simulink model "kalman_filter"  (Simulink 8.7)
settings: Solver=FixedStepAuto  StartTime=0.0  StopTime=10.0  FixedStep=dt  RelTol=1e-3
values from neighbouring files (symbols this model uses):
  A = [1 dt; 0 1]    [kalman_filter_init.m]
  B = zeros(2, 1)    [kalman_filter_init.m]
  dt = 1/50    (= 0.02)    [kalman_filter_init.m]
  H = eye(2, 2)    [kalman_filter_init.m]
  P0 = Q    [kalman_filter_init.m]
  Q = 0.01*eye(2,2)    [kalman_filter_init.m]
  R = 0.95*eye(2,2)    [kalman_filter_init.m]
  x0 = [0 0]'    [kalman_filter_init.m]
  x_seed = round(abs(rand()*1000))    [kalman_filter_init.m]
  xdot_seed = round(abs(rand()*1000))    [kalman_filter_init.m]
libraries: aerolibnav x2
settings Model: Creator=jason  LastModifiedBy=jason
settings DataIOCC: LimitDataPoints=off  SaveFormat=Dataset
settings DebuggingCC: UnderspecifiedInitializationDetection=Simplified  MergeDetectMultiDrivingBlocksExec=error
settings HardwareCC: ProdBitPerPointer=64  ProdLargestAtomicFloat=Float  ProdIntDivRoundTo=Zero  ProdEndianess=LittleEndian  ProdWordSize=64  ProdHWDeviceType=Intel->x86-64 (Windows64)
settings ModelReferenceCC: PropagateSignalLabelsOutOfModel=on
settings ConfigComp: CovModelRefEnable=off

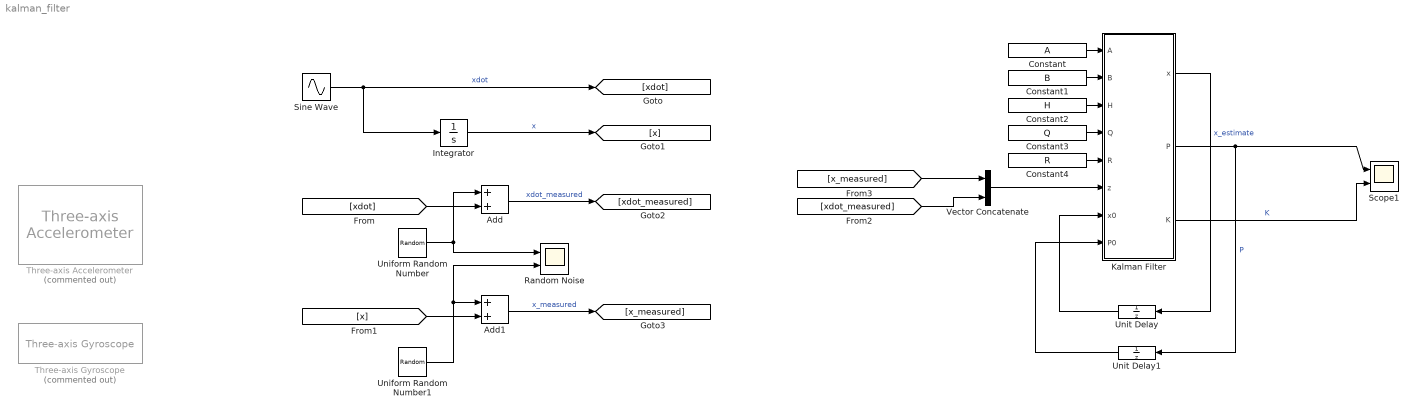
== system kalman_filter ==
  Add : Sum
  Add1 : Sum
  Constant : Constant  Value=A
  Constant1 : Constant  Value=B
  Constant2 : Constant  Value=H
  Constant3 : Constant  Value=Q
  Constant4 : Constant  Value=R
  Integrator : Integrator
  Kalman Filter : MATLAB Function  TreatAsAtomicUnit=on
  Random Noise : Scope  NumInputPorts=2
  Scope1 : Scope  NumInputPorts=2
  Sine Wave : Sin  SampleTime=0
  Three-axis Accelerometer : aerolibnav/Three-axis Accelerometer  Commented=on  units=Metric (MKS)  acc=[0 0 0]  gtype=on  dtype_a=on  w_a=190  z_a=0.707  a_sf_cc=[1 0 0; 0 1 0; 0 0 1]  a_bias=[0 0 0]  a_Ts=0  a_rand=on  a_seeds=[23093 23094 23095]  a_pow=[0.001 0.001 0.001]  a_sat="[-inf  -inf  -inf  inf inf inf]"
  Three-axis Gyroscope : aerolibnav/Three-axis Gyroscope  Commented=on  dtype_g=on  w_g=190  z_g=0.707  g_sf_cc=[1 0 0; 0 1 0; 0 0 1]  g_bias=[0 0 0]  g_sen=[0 0 0]  g_Ts=0  g_rand=on  g_seeds=[23093 23094 23095]  g_pow=[0.0001 0.0001 0.0001]  g_sat="[-inf  -inf  -inf  inf inf inf]"
  Uniform Random Number : UniformRandomNumber  Seed=xdot_seed  SampleTime=dt
  Uniform Random Number1 : UniformRandomNumber  Seed=x_seed  SampleTime=dt
  Unit Delay : UnitDelay  InitialCondition=x0  SampleTime=-1
  Unit Delay1 : UnitDelay  InitialCondition=P0  SampleTime=-1
  Vector Concatenate : Concatenate
  wires:
  Sine Wave/1 -> [xdot], Integrator/1  "xdot"
  Integrator/1 -> [x]  "x"
  [xdot] -> Add/2
  [x] -> Add1/2
  Uniform Random Number1/1 -> Add1/1, Random Noise/2
  Uniform Random Number/1 -> Add/1, Random Noise/1
  Add/1 -> [xdot_measured]  "xdot_measured"
  Add1/1 -> [x_measured]  "x_measured"
  Kalman Filter/2(P) -> Scope1/1, Unit Delay1/1  "P"
  Kalman Filter/1(x) -> Unit Delay/1  "x_estimate"
  Unit Delay/1 -> Kalman Filter/7(x0)
  Unit Delay1/1 -> Kalman Filter/8(P0)
  Vector Concatenate/1 -> Kalman Filter/6(z)
  [x_measured] -> Vector Concatenate/1
  [xdot_measured] -> Vector Concatenate/2
  Constant/1 -> Kalman Filter/1(A)
  Constant1/1 -> Kalman Filter/2(B)
  Constant3/1 -> Kalman Filter/4(Q)
  Constant2/1 -> Kalman Filter/3(H)
  Constant4/1 -> Kalman Filter/5(R)
  Kalman Filter/3(K) -> Scope1/2  "K"

== matlab function Kalman Filter ==
  data: A input double; B input double; H input double; Q input double; R input double; z input double; x0 input double; x output double; P0 input double; P output double; K output double
function [x, P, K] = fcn(A, B, H, Q, R, z, x0, P0)
%#codegen

[xp, Pp] = predict(A, Q, x0, P0);
[x, P, K] = correct(H, R, xp, z, Pp);

end

function [xp, Pp] = predict(A, Q, x0, P0)

xp = A*x0;
Pp = A*P0*A+Q;

end

function [x, P, K] = correct(H, R, xp, z, Pp)

[m,n] = size(Pp);

K = Pp*H'*inv(H*Pp*H'+R);
x = xp+K*(z-H*xp);
P = (eye(m,n)-K*H)*Pp;

end
